simulink model "gm_L3G4200D_SPI_interface"  (R2014b)
settings: Solver=FixedStepDiscrete  StartTime=0.0  StopTime=inf  FixedStep=.001  RelTol=1e-3
model workspace (MAT data in the model file):
  message_length = Simulink.Parameter
  message_length.Value = 16
  message_length.DataType = 'uint16'
  clk_freq = Simulink.Parameter
  clk_freq.Value = 1000000
  clk_freq.DataType = 'uint32'
  cs_to_clk_edge = Simulink.Parameter
  cs_to_clk_edge.Value = 10
  cs_to_clk_edge.DataType = 'uint16'
  stall_time = Simulink.Parameter
  stall_time.Value = 4
  stall_time.DataType = 'uint16'
undefined symbols (not defined in the file): AXI4, Lite
libraries: axiinterfacelib x8, simulink x3
settings Model: FPTRunName=FPA_Reference  SimulationMode=external  CovPath=/hdl_dut/Transmit  CovMetricSettings=re  CovHtmlReporting=off  CovReportOnPause=off  Creator=dlwalter  LastModifiedBy=dlwalter
settings SolverCC: PositivePriorityOrder=on
settings DataIOCC: SaveOutput=off  SaveTime=off
settings OptimizationCC: OptimizeModelRefInitCode=on  LifeSpan=1  MaxStackSize=64
settings DebuggingCC: UnderspecifiedInitializationDetection=Classic  MergeDetectMultiDrivingBlocksExec=none
settings HardwareCC: ProdLargestAtomicInteger=Long  ProdLargestAtomicFloat=Double  ProdEndianess=LittleEndian  ProdHWDeviceType=ARM Compatible->ARM Cortex  TargetLargestAtomicInteger=Long  TargetLargestAtomicFloat=Double  TargetIntDivRoundTo=Zero  TargetEndianess=LittleEndian  TargetHWDeviceType=ARMCortex  ProdEqTarget=off
settings RTWCC: SystemTargetFile=ert.tlc  TLCOptions=-aInlineSetEventsForThisBaseRateFcn=TLC_FALSE -aSuppressMultiTaskScheduler=TLC_FALSE  TemplateMakefile=ert_default_tmf  Description=Embedded Coder  ProcessScript=idelink_ert_make_rtw_hook  Toolchain=Xilinx ISE Design Suite 14.4
settings CodeAppCC: IgnoreCustomStorageClasses=off
settings ERTTargetCC: ParMdlRefBuildCompliant=off  GeneratePreprocessorConditionals=Disable all  CPPClassGenCompliant=off

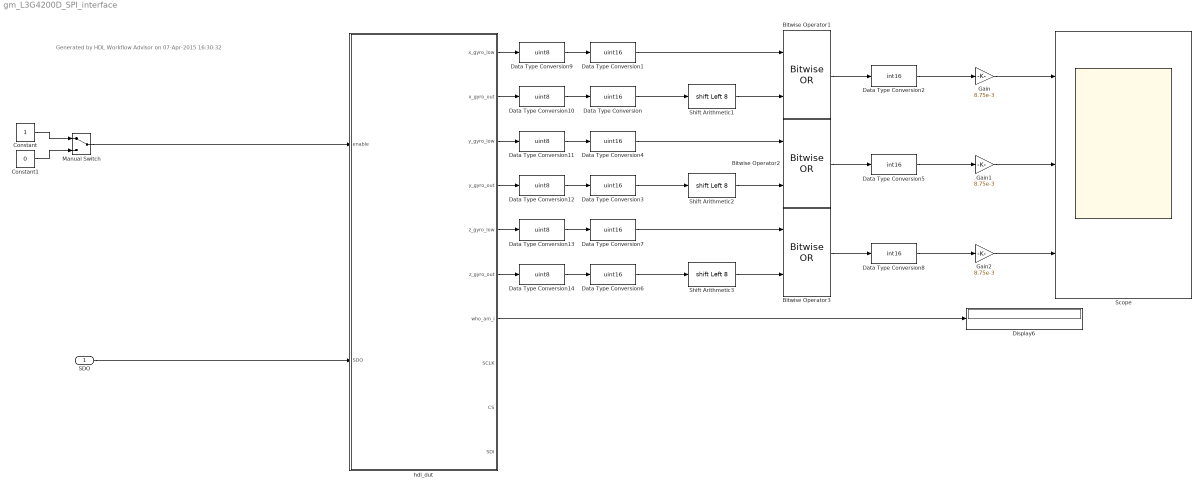
== system gm_L3G4200D_SPI_interface ==
  note: Generated by HDL Workflow Advisor on 07-Apr-2015 16:30:32
  SDO : Inport
  Bitwise Operator1 : simulink/Logic and Bit Operations/Bitwise Operator  logicop=OR  UseBitMask=off  NumInputPorts=2  BitMask=bin2dec('11011001')  BitMaskRealWorld=Stored Integer
  Bitwise Operator2 : simulink/Logic and Bit Operations/Bitwise Operator  logicop=OR  UseBitMask=off  NumInputPorts=2  BitMask=bin2dec('11011001')  BitMaskRealWorld=Stored Integer
  Bitwise Operator3 : simulink/Logic and Bit Operations/Bitwise Operator  logicop=OR  UseBitMask=off  NumInputPorts=2  BitMask=bin2dec('11011001')  BitMaskRealWorld=Stored Integer
  Constant : Constant  OutDataTypeStr=boolean  SampleTime=-1
  Constant1 : Constant  Value=0  OutDataTypeStr=boolean  SampleTime=-1
  Data Type Conversion{,1,3..4,6..7} (6 alike) : DataTypeConversion  OutDataTypeStr=uint16
  Data Type Conversion{9..14} (6 alike) : DataTypeConversion  OutDataTypeStr=uint8
  Data Type Conversion2 : DataTypeConversion  OutDataTypeStr=int16
  Data Type Conversion5 : DataTypeConversion  OutDataTypeStr=int16
  Data Type Conversion8 : DataTypeConversion  OutDataTypeStr=int16
  Display6 : Display
      settings: Format=binary (Stored Integer)
  Gain : Gain  Gain=8.75e-3
  Gain1 : Gain  Gain=8.75e-3
  Gain2 : Gain  Gain=8.75e-3
  Manual Switch : ManualSwitch
  Scope : Scope  NumInputPorts=3
      settings: TimeRange=1  YMin=-10~-10~-3000  YMax=10~10~3000
  Shift Arithmetic1 : ArithShift  BitShiftNumber=8  BitShiftDirection=Left
  Shift Arithmetic2 : ArithShift  BitShiftNumber=8  BitShiftDirection=Left
  Shift Arithmetic3 : ArithShift  BitShiftNumber=8  BitShiftDirection=Left
  hdl_dut : Subsystem  TreatAsAtomicUnit=on  MinMaxOverflowLogging=MinMaxAndOverflow  mask(AXI4-Lite/AXI4 Interface){}
      mask help:
      | This is an automatically generated subsystem block.
      | This contains the AXI4-Lite/AXI4 interface which communicates with the l3g4200d_spi_hdl_dut_pcore IPCore generated from L3G4200D_SPI/hdl_dut subsystem.
      mask Display: disp(sprintf('Xilinx Zynq \nAXI4-Lite/AXI4 Interface'));
  wires:
  Constant1/1 -> Manual Switch/2
  Constant/1 -> Manual Switch/1
  hdl_dut/7(who_am_i) -> Display6/1
  hdl_dut/5(z_gyro_low) -> Data Type Conversion13/1
  hdl_dut/6(z_gyro_out) -> Data Type Conversion14/1
  hdl_dut/4(y_gyro_out) -> Data Type Conversion12/1
  hdl_dut/3(y_gyro_low) -> Data Type Conversion11/1
  hdl_dut/2(x_gyro_out) -> Data Type Conversion10/1
  SDO/1 -> hdl_dut/2(SDO)
  Manual Switch/1 -> hdl_dut/1(enable)
  Data Type Conversion/1 -> Shift Arithmetic1/1
  Shift Arithmetic1/1 -> Bitwise Operator1/2
  hdl_dut/1(x_gyro_low) -> Data Type Conversion9/1
  Data Type Conversion1/1 -> Bitwise Operator1/1
  Bitwise Operator1/1 -> Data Type Conversion2/1
  Data Type Conversion2/1 -> Gain/1
  Data Type Conversion3/1 -> Shift Arithmetic2/1
  Shift Arithmetic2/1 -> Bitwise Operator2/2
  Data Type Conversion4/1 -> Bitwise Operator2/1
  Bitwise Operator2/1 -> Data Type Conversion5/1
  Data Type Conversion5/1 -> Gain1/1
  Data Type Conversion6/1 -> Shift Arithmetic3/1
  Shift Arithmetic3/1 -> Bitwise Operator3/2
  Data Type Conversion7/1 -> Bitwise Operator3/1
  Bitwise Operator3/1 -> Data Type Conversion8/1
  Data Type Conversion8/1 -> Gain2/1
  Gain/1 -> Scope/1
  Gain1/1 -> Scope/2
  Gain2/1 -> Scope/3
  Data Type Conversion9/1 -> Data Type Conversion1/1
  Data Type Conversion10/1 -> Data Type Conversion/1
  Data Type Conversion11/1 -> Data Type Conversion4/1
  Data Type Conversion12/1 -> Data Type Conversion3/1
  Data Type Conversion13/1 -> Data Type Conversion7/1
  Data Type Conversion14/1 -> Data Type Conversion6/1

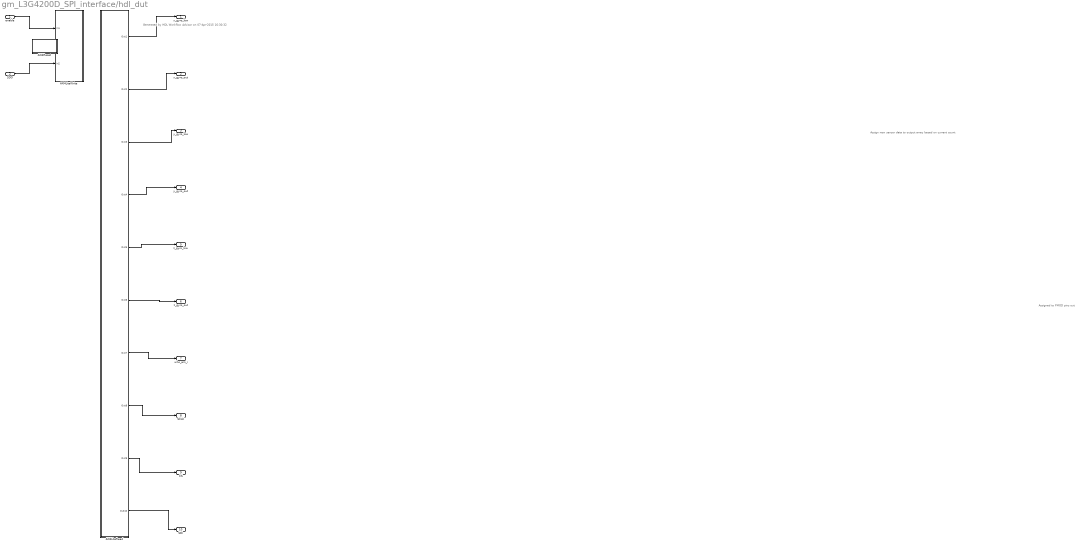
== system gm_L3G4200D_SPI_interface/hdl_dut ==
  note: Assigned to PMOD pins out
  note: Assign new sensor data to output array based on current count
  note: Generated by HDL Workflow Advisor on 07-Apr-2015 16:30:32
  enable : Inport
  SDO : Inport  Port=2
  AXI4LiteRead : Subsystem  Priority=10
  AXI4LiteWrite : Subsystem  Priority=1
  AXI4Reset : Subsystem  mask(System Initialize){ShowInLibBrowser=0}
      mask prompts: ShowInLibBrowser "Simulink:masks:CustCodeMaskParam1_MP"
      settings: CopyFcn=cccopyfcn(gcb)  OpenFcn=ccopenfcn('System Initialize Function')
      mask Help: eval('feval(''rtwprivate'',''rtwhelpview'',''rtw_sys_initialize_block'')');
      mask Display: disp('System\nInitialize');
  x_gyro_low : Outport
  x_gyro_out : Outport  Port=2
  y_gyro_low : Outport  Port=3
  y_gyro_out : Outport  Port=4
  z_gyro_low : Outport  Port=5
  z_gyro_out : Outport  Port=6
  who_am_i : Outport  Port=7
  SCLK : Outport  Port=8
  CS : Outport  Port=9
  SDI : Outport  Port=10
  wires:
  enable/1 -> AXI4LiteWrite/1(In1)
  SDO/1 -> AXI4LiteWrite/2(In2)
  AXI4LiteRead/1(Out1) -> x_gyro_low/1
  AXI4LiteRead/2(Out2) -> x_gyro_out/1
  AXI4LiteRead/3(Out3) -> y_gyro_low/1
  AXI4LiteRead/4(Out4) -> y_gyro_out/1
  AXI4LiteRead/5(Out5) -> z_gyro_low/1
  AXI4LiteRead/6(Out6) -> z_gyro_out/1
  AXI4LiteRead/7(Out7) -> who_am_i/1
  AXI4LiteRead/8(Out8) -> SCLK/1
  AXI4LiteRead/9(Out9) -> CS/1
  AXI4LiteRead/10(Out10) -> SDI/1

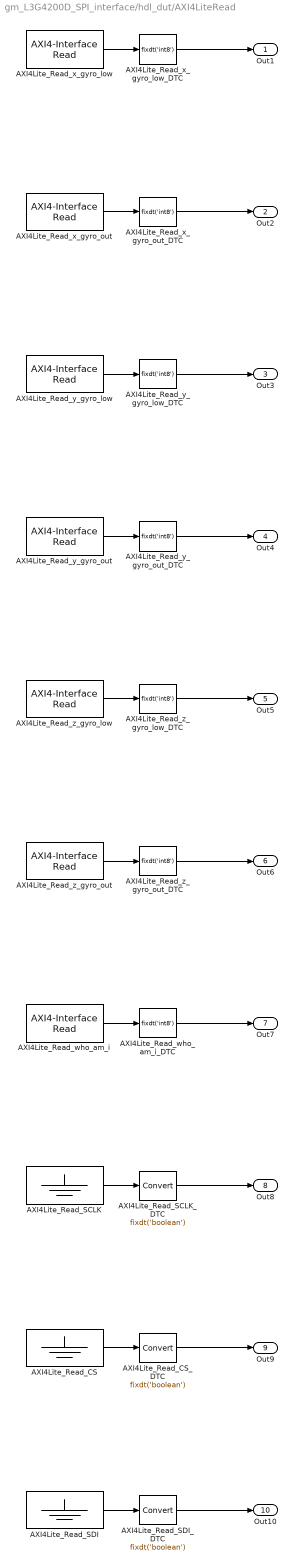
== system gm_L3G4200D_SPI_interface/hdl_dut/AXI4LiteRead ==
  AXI4Lite_Read_CS : Ground
  AXI4Lite_Read_CS_DTC : DataTypeConversion  OutDataTypeStr=fixdt('boolean')  ConvertRealWorld=Stored Integer (SI)
  AXI4Lite_Read_SCLK : Ground
  AXI4Lite_Read_SCLK_DTC : DataTypeConversion  OutDataTypeStr=fixdt('boolean')  ConvertRealWorld=Stored Integer (SI)
  AXI4Lite_Read_SDI : Ground
  AXI4Lite_Read_SDI_DTC : DataTypeConversion  OutDataTypeStr=fixdt('boolean')  ConvertRealWorld=Stored Integer (SI)
  AXI4Lite_Read_who_am_i : axiinterfacelib/AXI4-Interface Read  Priority=8  AXIInterfaceType=AXI4-Lite  DeviceName=/dev/mwipcore  RegisterOffset=hex2dec('11C')  DataType=uint32  DataLength=4096  SampleTime=-1  blockPlatform=ZYNQ  SimulateUsing=Interpreted Execution
  AXI4Lite_Read_who_am_i_DTC : DataTypeConversion  OutDataTypeStr=fixdt('int8')  ConvertRealWorld=Stored Integer (SI)
  AXI4Lite_Read_x_gyro_low : axiinterfacelib/AXI4-Interface Read  Priority=2  AXIInterfaceType=AXI4-Lite  DeviceName=/dev/mwipcore  RegisterOffset=hex2dec('104')  DataType=uint32  DataLength=4096  SampleTime=-1  blockPlatform=ZYNQ  SimulateUsing=Interpreted Execution
  AXI4Lite_Read_x_gyro_low_DTC : DataTypeConversion  OutDataTypeStr=fixdt('int8')  ConvertRealWorld=Stored Integer (SI)
  AXI4Lite_Read_x_gyro_out : axiinterfacelib/AXI4-Interface Read  Priority=3  AXIInterfaceType=AXI4-Lite  DeviceName=/dev/mwipcore  RegisterOffset=hex2dec('108')  DataType=uint32  DataLength=4096  SampleTime=-1  blockPlatform=ZYNQ  SimulateUsing=Interpreted Execution
  AXI4Lite_Read_x_gyro_out_DTC : DataTypeConversion  OutDataTypeStr=fixdt('int8')  ConvertRealWorld=Stored Integer (SI)
  AXI4Lite_Read_y_gyro_low : axiinterfacelib/AXI4-Interface Read  Priority=4  AXIInterfaceType=AXI4-Lite  DeviceName=/dev/mwipcore  RegisterOffset=hex2dec('10C')  DataType=uint32  DataLength=4096  SampleTime=-1  blockPlatform=ZYNQ  SimulateUsing=Interpreted Execution
  AXI4Lite_Read_y_gyro_low_DTC : DataTypeConversion  OutDataTypeStr=fixdt('int8')  ConvertRealWorld=Stored Integer (SI)
  AXI4Lite_Read_y_gyro_out : axiinterfacelib/AXI4-Interface Read  Priority=5  AXIInterfaceType=AXI4-Lite  DeviceName=/dev/mwipcore  RegisterOffset=hex2dec('110')  DataType=uint32  DataLength=4096  SampleTime=-1  blockPlatform=ZYNQ  SimulateUsing=Interpreted Execution
  AXI4Lite_Read_y_gyro_out_DTC : DataTypeConversion  OutDataTypeStr=fixdt('int8')  ConvertRealWorld=Stored Integer (SI)
  AXI4Lite_Read_z_gyro_low : axiinterfacelib/AXI4-Interface Read  Priority=6  AXIInterfaceType=AXI4-Lite  DeviceName=/dev/mwipcore  RegisterOffset=hex2dec('114')  DataType=uint32  DataLength=4096  SampleTime=-1  blockPlatform=ZYNQ  SimulateUsing=Interpreted Execution
  AXI4Lite_Read_z_gyro_low_DTC : DataTypeConversion  OutDataTypeStr=fixdt('int8')  ConvertRealWorld=Stored Integer (SI)
  AXI4Lite_Read_z_gyro_out : axiinterfacelib/AXI4-Interface Read  Priority=7  AXIInterfaceType=AXI4-Lite  DeviceName=/dev/mwipcore  RegisterOffset=hex2dec('118')  DataType=uint32  DataLength=4096  SampleTime=-1  blockPlatform=ZYNQ  SimulateUsing=Interpreted Execution
  AXI4Lite_Read_z_gyro_out_DTC : DataTypeConversion  OutDataTypeStr=fixdt('int8')  ConvertRealWorld=Stored Integer (SI)
  Out1 : Outport
  Out2 : Outport  Port=2
  Out3 : Outport  Port=3
  Out4 : Outport  Port=4
  Out5 : Outport  Port=5
  Out6 : Outport  Port=6
  Out7 : Outport  Port=7
  Out8 : Outport  Port=8
  Out9 : Outport  Port=9
  Out10 : Outport  Port=10
  wires:
  AXI4Lite_Read_y_gyro_out_DTC/1 -> Out4/1
  AXI4Lite_Read_y_gyro_low_DTC/1 -> Out3/1
  AXI4Lite_Read_y_gyro_low/1 -> AXI4Lite_Read_y_gyro_low_DTC/1
  AXI4Lite_Read_y_gyro_out/1 -> AXI4Lite_Read_y_gyro_out_DTC/1
  AXI4Lite_Read_z_gyro_low/1 -> AXI4Lite_Read_z_gyro_low_DTC/1
  AXI4Lite_Read_z_gyro_out_DTC/1 -> Out6/1
  AXI4Lite_Read_z_gyro_low_DTC/1 -> Out5/1
  AXI4Lite_Read_z_gyro_out/1 -> AXI4Lite_Read_z_gyro_out_DTC/1
  AXI4Lite_Read_who_am_i/1 -> AXI4Lite_Read_who_am_i_DTC/1
  AXI4Lite_Read_SCLK/1 -> AXI4Lite_Read_SCLK_DTC/1
  AXI4Lite_Read_SCLK_DTC/1 -> Out8/1
  AXI4Lite_Read_who_am_i_DTC/1 -> Out7/1
  AXI4Lite_Read_CS_DTC/1 -> Out9/1
  AXI4Lite_Read_SDI_DTC/1 -> Out10/1
  AXI4Lite_Read_CS/1 -> AXI4Lite_Read_CS_DTC/1
  AXI4Lite_Read_SDI/1 -> AXI4Lite_Read_SDI_DTC/1
  AXI4Lite_Read_x_gyro_low/1 -> AXI4Lite_Read_x_gyro_low_DTC/1
  AXI4Lite_Read_x_gyro_low_DTC/1 -> Out1/1
  AXI4Lite_Read_x_gyro_out_DTC/1 -> Out2/1
  AXI4Lite_Read_x_gyro_out/1 -> AXI4Lite_Read_x_gyro_out_DTC/1

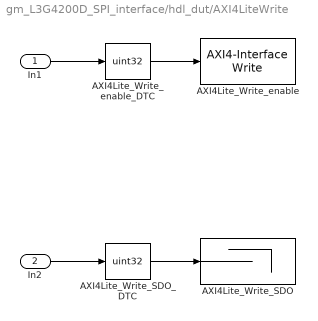
== system gm_L3G4200D_SPI_interface/hdl_dut/AXI4LiteWrite ==
  In1 : Inport
  In2 : Inport  Port=2
  AXI4Lite_Write_SDO : Terminator
  AXI4Lite_Write_SDO_DTC : DataTypeConversion  OutDataTypeStr=uint32  ConvertRealWorld=Stored Integer (SI)
  AXI4Lite_Write_enable : axiinterfacelib/AXI4-Interface Write  Priority=1  AXIInterfaceType=AXI4-Lite  DeviceName=/dev/mwipcore  RegisterOffset=hex2dec('100')  blockPlatform=ZYNQ  SimulateUsing=Interpreted execution
  AXI4Lite_Write_enable_DTC : DataTypeConversion  OutDataTypeStr=uint32  ConvertRealWorld=Stored Integer (SI)
  wires:
  AXI4Lite_Write_enable_DTC/1 -> AXI4Lite_Write_enable/1
  In1/1 -> AXI4Lite_Write_enable_DTC/1
  In2/1 -> AXI4Lite_Write_SDO_DTC/1
  AXI4Lite_Write_SDO_DTC/1 -> AXI4Lite_Write_SDO/1

== system gm_L3G4200D_SPI_interface/hdl_dut/AXI4Reset ==
